simulink model "PID_digital_tarea"  (R2014a)
settings: Solver=ode45  StartTime=0.0  StopTime=5  MaxStep=1e-5  RelTol=1e-3
undefined symbols (not defined in the file or in its folder): DiscIntNeverNeededParam
libraries: simulink x1
settings Model: Creator=Usuario  LastModifiedBy=Ernesto
settings DataIOCC: LimitDataPoints=off  SignalLoggingSaveFormat=ModelDataLogs
settings OptimizationCC: InitFltsAndDblsToZero=on
settings DebuggingCC: SaveWithParameterizedLinksMsg=none  UnderspecifiedInitializationDetection=Classic  SignalResolutionControl=TryResolveAllWithWarning  MultiTaskDSMMsg=warning  MultiTaskCondExecSysMsg=none  FcnCallInpInsideContextMsg=UseLocalSettings
settings RTWCC: IncludeERTFirstTime=on
settings GRTTargetCC: TargetFcnLib=ansi_tfl_tmw.mat  CombineOutputUpdateFcns=off  GRTInterface=on

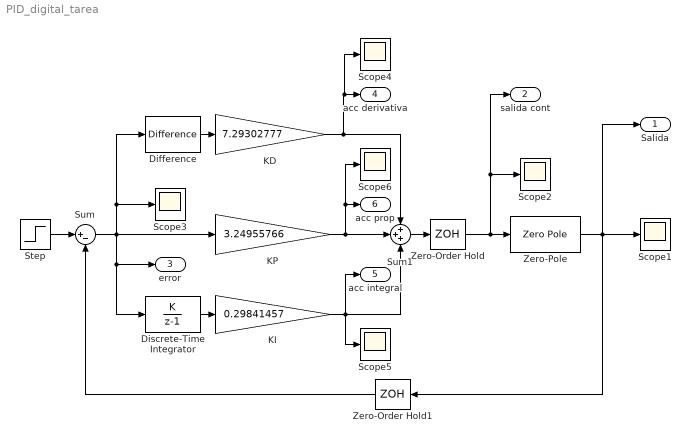
== system PID_digital_tarea ==
  Difference : simulink/Discrete/Difference  ICPrevInput=0.0  InputProcessing=Inherited  OutMin=[]  OutMax=[]  OutDataType=fixdt(1, 16)  OutScaling=2^-10  DoSatur=off
  Discrete-Time Integrator : DiscreteIntegrator  IntegratorMethod=Accumulation: Forward Euler  SampleTime=-1  ICPrevOutput=DiscIntNeverNeededParam  ICPrevScaledInput=DiscIntNeverNeededParam
  KD : Gain  Gain=7.29302777
  KI : Gain  Gain=0.29841457
  KP : Gain  Gain=3.24955766
  Scope{1..6} (6 alike) : Scope
      Scope1 settings: ShowLegends=on  YMin=0.96  YMax=1.03  SampleInput=on
      Scope2 settings: ShowLegends=on  YMin=0.599998  YMax=0.6  SampleInput=on
      Scope3 settings: ShowLegends=on  YMin=0.96  YMax=1.03  SaveName=ScopeData5  SampleInput=on
      Scope4 settings: ShowLegends=on  YMin=0.96  YMax=1.03  SaveName=ScopeData2  SampleInput=on
      Scope5 settings: ShowLegends=on  YMin=0.96  YMax=1.03  SaveName=ScopeData4  SampleInput=on
      Scope6 settings: ShowLegends=on  YMin=0.96  YMax=1.03  SaveName=ScopeData3  SampleInput=on
  Step : Step  Time=0  SampleTime=0.07
  Sum : Sum  Inputs=|+-
  Sum1 : Sum  Inputs=+++
  Zero-Order Hold : ZeroOrderHold  SampleTime=0.07
  Zero-Order Hold1 : ZeroOrderHold  SampleTime=0.07
  Zero-Pole : ZeroPole  Zeros=[]  Poles=[-2 -3]  Gain=[10]
  Salida : Outport
  salida cont : Outport  Port=2
  error : Outport  Port=3
  acc derivativa : Outport  Port=4
  acc integral : Outport  Port=5
  acc prop : Outport  Port=6
  wires:
  Step/1 -> Sum/1
  Zero-Pole/1 -> Salida/1, Zero-Order Hold1/1, Scope1/1
  KI/1 -> Scope5/1, Sum1/3, acc integral/1
  KP/1 -> Sum1/2, Scope6/1, acc prop/1
  Zero-Order Hold1/1 -> Sum/2
  Sum1/1 -> Zero-Order Hold/1
  KD/1 -> Scope4/1, acc derivativa/1, Sum1/1
  Difference/1 -> KD/1
  Discrete-Time Integrator/1 -> KI/1
  Sum/1 -> error/1, Discrete-Time Integrator/1, Scope3/1, Difference/1, KP/1
  Zero-Order Hold/1 -> Zero-Pole/1, Scope2/1, salida cont/1
